simulink model "sim2el17128"  (R2019b)
settings: Solver=ode45  StartTime=0.0  StopTime=10  MaxStep=1e-4  RelTol=1e-3
values from neighbouring files (symbols this model uses):
  b1 = 0.1796    [scriptsim2el17128.m]
  b2 = 0.0012    [scriptsim2el17128.m]
  f1 = 50    [scriptsim2el17128.m]
  f2 = 25    [scriptsim2el17128.m]
  J = 0.08    [scriptsim2el17128.m]
  K = 1/sqrt(2)    [scriptsim2el17128.m]
  LM = 0.1237    [scriptsim2el17128.m]
  Lsigma = 0.0227    [scriptsim2el17128.m]
  np = 2    [scriptsim2el17128.m]
  RR = 0.8197    [scriptsim2el17128.m]
  Rs = 2.2667    [scriptsim2el17128.m]
  sw1 = 1    [scriptsim2el17128.m]
  sw2 = 1    [scriptsim2el17128.m]
  sw3 = 0    [scriptsim2el17128.m]
  tL = 26.8    [scriptsim2el17128.m]
  Vn = 230*sqrt(2)    [scriptsim2el17128.m]
  wbase = 314.15    [scriptsim2el17128.m]
undefined symbols (not defined in the file or in its folder): magnitude
settings Model: Creator=user  LastModifiedBy=user

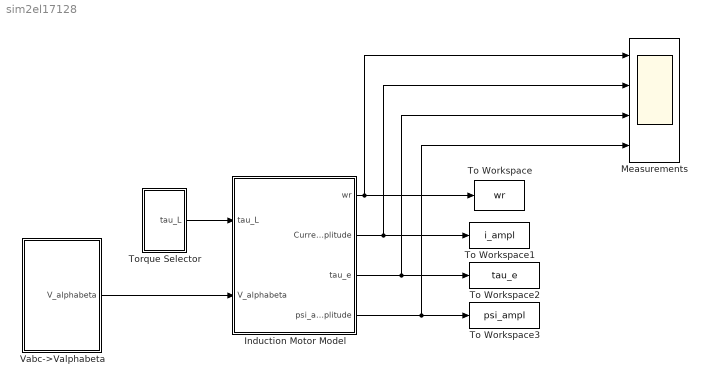
== system sim2el17128 ==
  Induction Motor Model : Subsystem
  Measurements : Scope  NumInputPorts=4
  To Workspace : ToWorkspace  VariableName=wr  SaveFormat=Structure With Time  SampleTime=-1
  To Workspace1 : ToWorkspace  VariableName=i_ampl  SaveFormat=Structure With Time  SampleTime=-1
  To Workspace2 : ToWorkspace  VariableName=tau_e  SaveFormat=Structure With Time  SampleTime=-1
  To Workspace3 : ToWorkspace  VariableName=psi_ampl  SaveFormat=Structure With Time  SampleTime=-1
  Torque Selector : Subsystem
  Vabc->Valphabeta : Subsystem
  wires:
  Vabc->Valphabeta/1(V_alphabeta) -> Induction Motor Model/2(V_alphabeta)
  Induction Motor Model/1(wr) -> Measurements/1, To Workspace/1
  Induction Motor Model/3(tau_e) -> Measurements/3, To Workspace2/1
  Induction Motor Model/2(Current amplitude) -> Measurements/2, To Workspace1/1
  Induction Motor Model/4(psi_amplitude) -> Measurements/4, To Workspace3/1
  Torque Selector/1(tau_L) -> Induction Motor Model/1(tau_L)

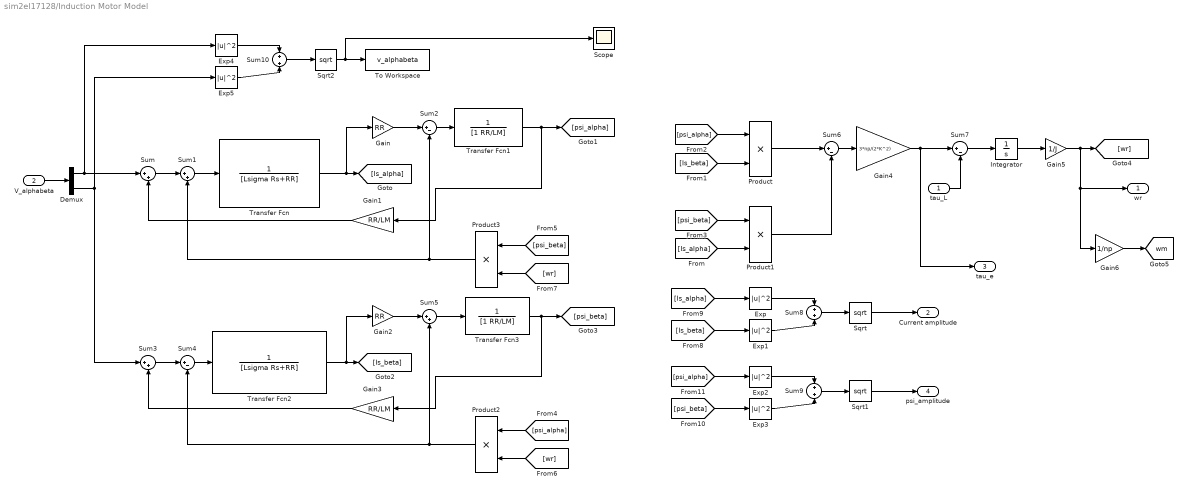
== system sim2el17128/Induction Motor Model ==
  tau_L : Inport
  V_alphabeta : Inport  Port=2
  Demux : Demux  Outputs=2
  Exp{,1..5} (6 alike) : Math  Operator=magnitude^2  SignedPower=off  SaturateOnIntegerOverflow=on
  Gain : Gain  Gain=RR
  Gain1 : Gain  Gain=RR/LM
  Gain2 : Gain  Gain=RR
  Gain3 : Gain  Gain=RR/LM
  Gain4 : Gain  Gain=3*np/(2*K^2)
  Gain5 : Gain  Gain=1/J
  Gain6 : Gain  Gain=1/np
  Integrator : Integrator
  Product{,1..3} (4 alike) : Product
  Scope : Scope
  Sqrt : Sqrt  SaturateOnIntegerOverflow=on
  Sqrt1 : Sqrt  SaturateOnIntegerOverflow=on
  Sqrt2 : Sqrt  SaturateOnIntegerOverflow=on
  Sum{,1,3,5} (4 alike) : Sum  Inputs=|++
  Sum10 : Sum  Inputs=+|+
  Sum{2,4,6..7} (4 alike) : Sum  Inputs=|+-
  Sum8 : Sum  Inputs=+|+
  Sum9 : Sum  Inputs=+|+
  To Workspace : ToWorkspace  VariableName=v_alphabeta  SaveFormat=Timeseries  SampleTime=-1
  Transfer Fcn : TransferFcn  Denominator=[Lsigma Rs+RR]
  Transfer Fcn1 : TransferFcn  Denominator=[1 RR/LM]
  Transfer Fcn2 : TransferFcn  Denominator=[Lsigma Rs+RR]
  Transfer Fcn3 : TransferFcn  Denominator=[1 RR/LM]
  wr : Outport
  Current amplitude : Outport  Port=2
  tau_e : Outport  Port=3
  psi_amplitude : Outport  Port=4
  tag scope: wm=global
  wires:
  Transfer Fcn1/1 -> Gain1/1, [psi_alpha]
  Product3/1 -> Sum1/2, Sum2/2
  Product2/1 -> Sum4/2, Sum5/2
  [Is_beta] -> Exp1/1
  Gain5/1 -> Gain6/1, wr/1, [wr]
  [Is_beta] -> Product/2
  Product/1 -> Sum6/1
  [wr] -> Product2/2
  Sqrt/1 -> Current amplitude/1
  Sum3/1 -> Sum4/1
  Transfer Fcn3/1 -> Gain3/1, [psi_beta]
  [psi_beta] -> Product1/1
  Sum5/1 -> Transfer Fcn3/1
  Transfer Fcn2/1 -> Gain2/1, [Is_beta]
  Sum1/1 -> Transfer Fcn/1
  V_alphabeta/1 -> Demux/1
  [Is_alpha] -> Product1/2
  Gain1/1 -> Sum/2
  Demux/2 -> Exp5/1, Sum3/1
  Demux/1 -> Exp4/1, Sum/1
  Exp/1 -> Sum8/1
  tau_L/1 -> Sum7/2
  Sum/1 -> Sum1/1
  Sum6/1 -> Gain4/1
  Gain4/1 -> tau_e/1, Sum7/1
  Transfer Fcn/1 -> Gain/1, [Is_alpha]
  [psi_alpha] -> Product/1
  Sum2/1 -> Transfer Fcn1/1
  Gain3/1 -> Sum3/2
  Gain2/1 -> Sum5/1
  Sum4/1 -> Transfer Fcn2/1
  Product1/1 -> Sum6/2
  [Is_alpha] -> Exp/1
  Sum8/1 -> Sqrt/1
  Gain/1 -> Sum2/1
  [wr] -> Product3/2
  [psi_beta] -> Product3/1
  Sum7/1 -> Integrator/1
  Integrator/1 -> Gain5/1
  [psi_alpha] -> Product2/1
  Exp1/1 -> Sum8/2
  Sum9/1 -> Sqrt1/1
  [psi_alpha] -> Exp2/1
  Exp3/1 -> Sum9/2
  [psi_beta] -> Exp3/1
  Exp2/1 -> Sum9/1
  Sqrt1/1 -> psi_amplitude/1
  Gain6/1 -> [wm]
  Exp5/1 -> Sum10/2
  Sum10/1 -> Sqrt2/1
  Exp4/1 -> Sum10/1
  Sqrt2/1 -> To Workspace/1, Scope/1

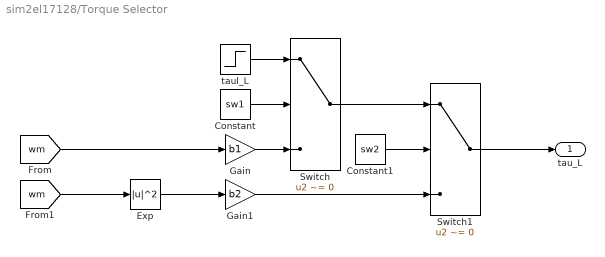
== system sim2el17128/Torque Selector ==
  Constant : Constant  Value=sw1
  Constant1 : Constant  Value=sw2
  Exp : Math  Operator=magnitude^2  SignedPower=off  SaturateOnIntegerOverflow=on
  Gain : Gain  Gain=b1
  Gain1 : Gain  Gain=b2
  Switch : Switch  Criteria=u2 ~= 0
  Switch1 : Switch  Criteria=u2 ~= 0
  taul_L : Step  Time=5  After=tL  SampleTime=0
  tau_L : Outport
  wires:
  Constant1/1 -> Switch1/2
  Constant/1 -> Switch/2
  Gain/1 -> Switch/3
  [wm] -> Gain/1
  Gain1/1 -> Switch1/3
  taul_L/1 -> Switch/1
  Switch/1 -> Switch1/1
  Switch1/1 -> tau_L/1
  Exp/1 -> Gain1/1
  [wm] -> Exp/1

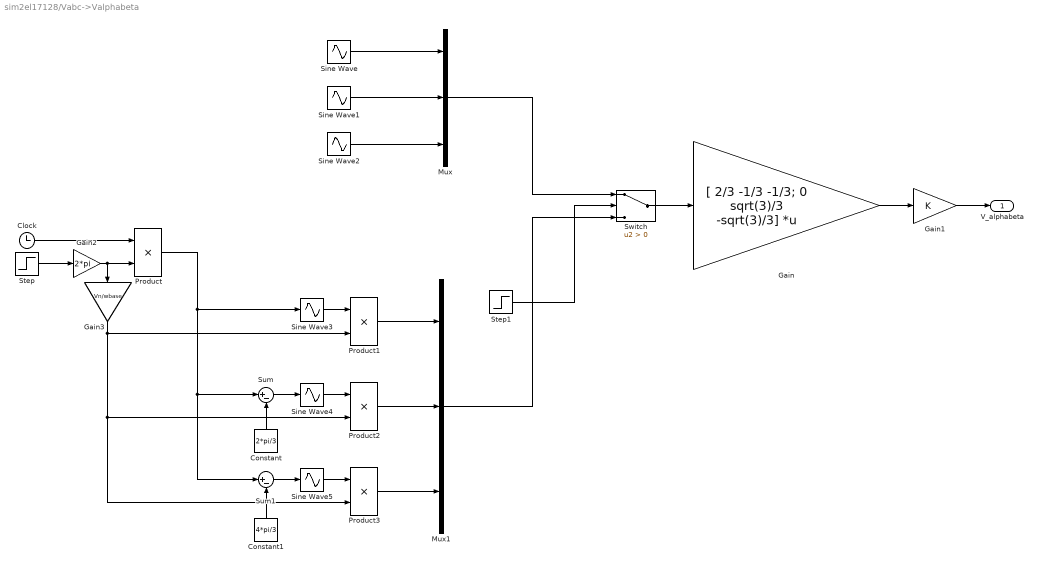
== system sim2el17128/Vabc->Valphabeta ==
  Clock : Clock
  Constant : Constant  Value=2*pi/3
  Constant1 : Constant  Value=4*pi/3
  Gain : Gain  Gain="[ 2/3   -1/3   -1/3; 0   sqrt(3)/3   -sqrt(3)/3]"  Multiplication=Matrix(K*u) (u vector)
  Gain1 : Gain  Gain=K
  Gain2 : Gain  Gain=2*pi
  Gain3 : Gain  Gain=Vn/wbase
  Mux : Mux  Inputs=3
  Mux1 : Mux  Inputs=3
  Product{,1..3} (4 alike) : Product
  Sine Wave : Sin  Amplitude=Vn  Frequency=314.1592  SampleTime=0
  Sine Wave1 : Sin  Amplitude=Vn  Frequency=314.1592  Phase=-2*pi/3  SampleTime=0
  Sine Wave2 : Sin  Amplitude=Vn  Frequency=314.1592  Phase=-4*pi/3  SampleTime=0
  Sine Wave3 : Sin  TimeSource=Use external signal  SampleTime=0
  Sine Wave4 : Sin  TimeSource=Use external signal  SampleTime=0
  Sine Wave5 : Sin  TimeSource=Use external signal  SampleTime=0
  Step : Step  Time=2.5  Before=f1  After=f2  SampleTime=0
  Step1 : Step  Time=0  Before=1  After=sw3  SampleTime=0
  Sum : Sum  Inputs=|+-
  Sum1 : Sum  Inputs=|+-
  Switch : Switch  Criteria=u2 > Threshold
  V_alphabeta : Outport
  wires:
  Sine Wave/1 -> Mux/1
  Sine Wave1/1 -> Mux/2
  Sine Wave2/1 -> Mux/3
  Gain/1 -> Gain1/1
  Clock/1 -> Product/1
  Product/1 -> Sum1/1, Sum/1, Sine Wave3/1
  Sum/1 -> Sine Wave4/1
  Sum1/1 -> Sine Wave5/1
  Constant/1 -> Sum/2
  Constant1/1 -> Sum1/2
  Mux/1 -> Switch/1
  Mux1/1 -> Switch/3
  Switch/1 -> Gain/1
  Gain1/1 -> V_alphabeta/1
  Step1/1 -> Switch/2
  Gain2/1 -> Product/2, Gain3/1
  Step/1 -> Gain2/1
  Product1/1 -> Mux1/1
  Sine Wave3/1 -> Product1/1
  Gain3/1 -> Product1/2, Product3/2, Product2/2
  Sine Wave4/1 -> Product2/1
  Product2/1 -> Mux1/2
  Product3/1 -> Mux1/3
  Sine Wave5/1 -> Product3/1
